simulink model "sim_2018"  (R2018a)
settings: Solver=ode4  StartTime=0.0  StopTime=31*60  FixedStep=0.001  RelTol=1e-3
model workspace: external: MAT-File E:\college\Sinior 2\2022\AutoPilot\task8\prameters.mat (data not in the file)
values from neighbouring files (symbols this model uses):
  g = aircraft_data(52)    [TF.m]    (also in param_code.m)
  IC = s0    [TF.m]    (also in param_code.m)
  Ixx = aircraft_data(53)    [TF.m]    (also in param_code.m)
  Iyy = aircraft_data(54)    [TF.m]    (also in param_code.m)
  Izz = aircraft_data(55)    [TF.m]    (also in param_code.m)
  m = aircraft_data(51)    [TF.m]    (also in param_code.m)
  mg0 = m*g * [ sin(s0(8)) ; -cos(s0(8))*sin(s0(7)) ; -cos(s0(8))*cos(s0(7)) ]    [TF.m]    (also in param_code.m)
  s0 = aircraft_data(4:15)    [TF.m]    (also in param_code.m)
  sdot0 = zeros(12,1)    [param_code.m]
  servo = tf(10,[1 10])    [TF.m]    (also in param_code.m)
  stability_matrix = [XU 0 XW 0 0 0 0 0 0 XDE XDTH;     0 U_Yv 0 Yp 0 Yr 0 U_Yda U_Ydr 0 0;     ZU 0 ZW 0 ZQ 0 ZWD 0 0 ZDE ZDTH;     0 U_Lv 0 U_Lp 0 U_Lr 0 U_Lda U_Ldr 0 0;     MU 0 MW 0 MQ 0 MWD 0 0 MDE MDTH;     0 U_Nv 0 U_Np 0 U_Nr 0 U_Nda U_Ndr 0 0]    [param_code.m]
  TH0 = s0(8)    [TF.m]    (also in param_code.m)
  U0 = s0(1)    [TF.m]    (also in param_code.m)
  W0 = s0(3)    [TF.m]    (also in param_code.m)
  z0 = s0(12)    [TF.m]    (also in param_code.m)
undefined symbols (not defined in the file or in its folder): rotationVectorToMatrix, sigbuilder_block
libraries: cstblocks x5, simulink_extras x3, shared6dof x1, sharedtransform x1, dspsigops x1
settings Model: Creator=engmh  LastModifiedBy=engmh

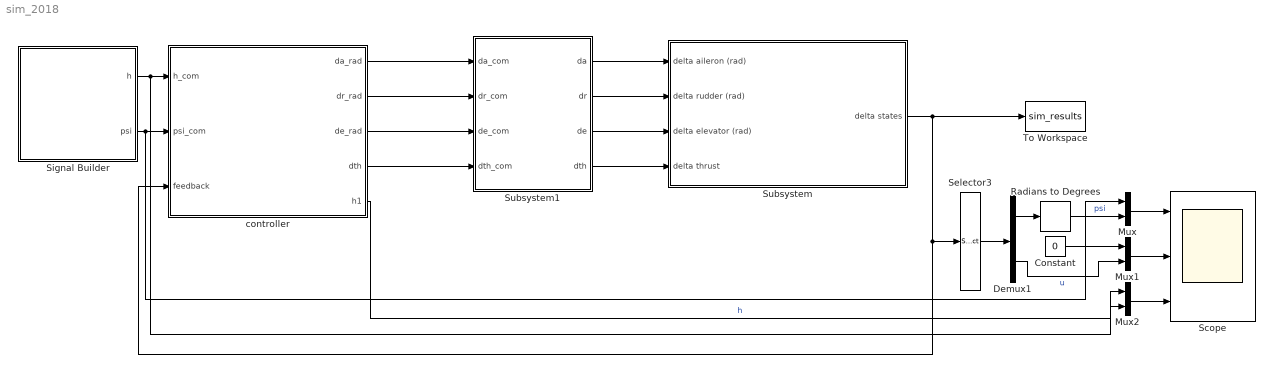
== system sim_2018 ==
  Constant : Constant  Value=0
  Demux1 : Demux  Outputs=2
  Mux : Mux  Inputs=2
  Mux1 : Mux  Inputs=2
  Mux2 : Mux  Inputs=2
  Radians to Degrees : simulink_extras/Transformations/Radians to Degrees
  Scope : Scope  NumInputPorts=3
  Selector3 : Selector  InputPortWidth=15  IndexOptions=Index vector (dialog)  Indices=[6 7 ]  OutputSizes=1
  Signal Builder : Subsystem  Tag=STV Subsys  LoadFcn=sigbuilder_block('load');  StartFcn=sigbuilder_block('start');  StopFcn=sigbuilder_block('stop');  ClipboardFcn=sigbuilder_block('clipboard');  mask(Sigbuilder block){tuvar=[0:10]}
      mask help: Simulink:masks:SigbuilderBlock_MD
      mask init:
      | if ~strcmp(get_param(bdroot(gcbh),'SimulationStatus'),'stopped') tuvar = sigbuilder_block('maskInit'); end
      settings: CopyFcn=sigbuilder_block('copy');  DeleteFcn=sigbuilder_block('delete');  ModelCloseFcn=sigbuilder_block('modelClose');  PreSaveFcn=sigbuilder_block('preSave');  PauseFcn=sigbuilder_block('pause');  ContinueFcn=sigbuilder_block('continue');  NameChangeFcn=sigbuilder_block('namechange');  OpenFcn=sigbuilder_block('open',[288.6 49.2 550.8 400.2 ]);  CloseFcn=sigbuilder_block('close');
      mask Display: plot(0, 0, 100, 100,[2, 2, 32, 32, 2], [68, 8, 8, 68, 68],[32, 2], [38, 38], [32, 19, 2],[53, 60, 44], [32, 17, 17, 2],[16, 16, 31, 31]);txt = getActiveGroup(gcbh);text(2, 100, txt,'verticalAlignment', 'top');
  Subsystem : Subsystem
  Subsystem1 : Subsystem
  To Workspace : ToWorkspace  VariableName=sim_results  SaveFormat=Timeseries  SampleTime=-1
  controller : Subsystem
  wires:
  Subsystem/1("delta states ") -> controller/3("feedback "), Selector3/1, To Workspace/1
  Subsystem1/1(da) -> Subsystem/1("delta aileron (rad) ")
  Subsystem1/2(dr) -> Subsystem/2(delta rudder (rad))
  Subsystem1/3(de) -> Subsystem/3(delta elevator (rad))
  Subsystem1/4(dth) -> Subsystem/4(delta thrust)
  Selector3/1 -> Demux1/1
  Demux1/1 -> Radians to Degrees/1
  Demux1/2 -> Mux1/2  "u"
  controller/1(da_rad) -> Subsystem1/1("da_com ")
  controller/2(dr_rad) -> Subsystem1/2(dr_com)
  controller/3(de_rad) -> Subsystem1/3(de_com)
  controller/4(dth) -> Subsystem1/4("dth_com ")
  controller/5("h1 ") -> Mux2/2  "h"
  Radians to Degrees/1 -> Mux/2  "psi"
  Signal Builder/2(psi) -> Mux/1, controller/2(psi_com)
  Signal Builder/1(h) -> Mux2/1, controller/1(h_com)
  Mux/1 -> Scope/1
  Mux1/1 -> Scope/2
  Mux2/1 -> Scope/3
  Constant/1 -> Mux1/1

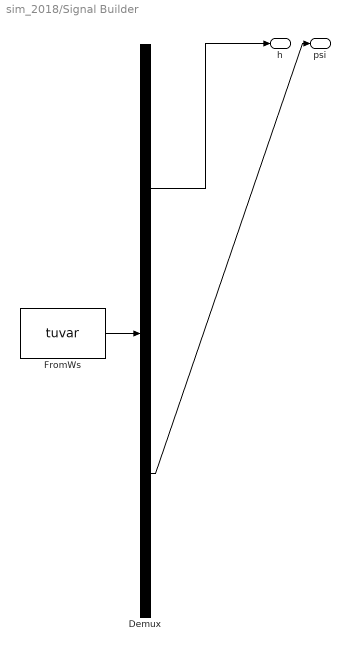
== system sim_2018/Signal Builder ==
  Demux : Demux  Tag=STV Demux  Outputs=2
  FromWs : FromWorkspace  Tag=STV FromWs  VariableName=tuvar  SampleTime=0
      SigBuilderData=|
      | common.afterFinalStr = 'Extrapolate'
      | common.sampleTime = 0
      | dataSet.timeRange = [0 1860]
      | dataSet.name = 'Group 1'
      | sbobj.Groups.Name = 'Group 1'
      | sbobj.Groups.Signals(1).Name = 'h'
      | sbobj.Groups.Signals(1).XData = [0 600 1080 1080 1200 1800 1860]
      | sbobj.Groups.Signals(1).YData = [0 10000 10000 10100 10100 0 0]
      | sbobj.Groups.Signals(2).Name = 'psi'
      | sbobj.Groups.Signals(2).XData = [0 720 720 1080 1080 1860]
      | sbobj.Groups.Signals(2).YData = [0 0 360 360 390 390]
      | sbobj.Groups.TimeRange = [0 1860]
  h : Outport  Tag=STV Outport
  psi : Outport  Tag=STV Outport  Port=2
  wires:
  Demux/1 -> h/1
  FromWs/1 -> Demux/1
  Demux/2 -> psi/1

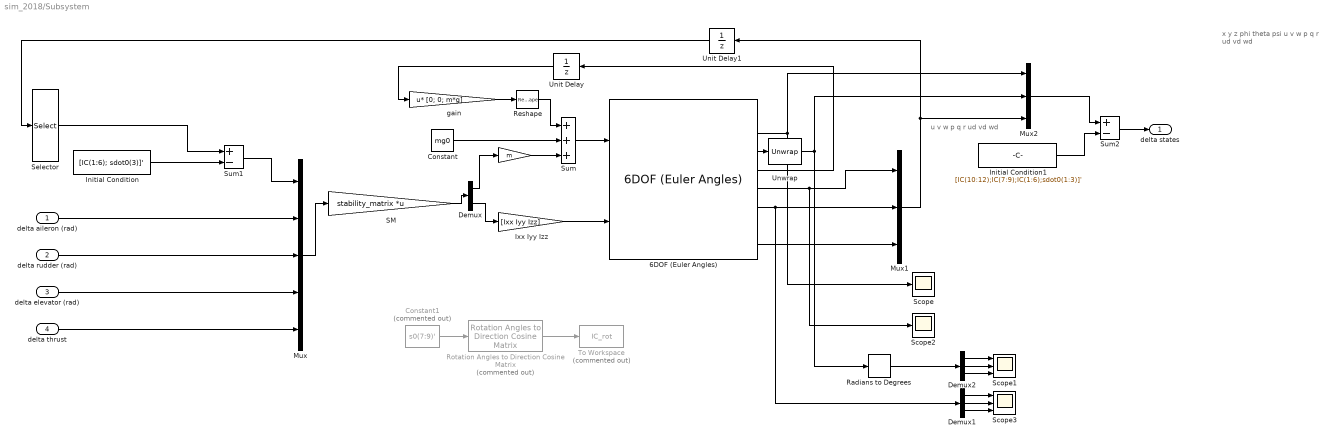
== system sim_2018/Subsystem ==
  note: u
      | v
      | w
      |
      | p
      | q
      | r
      |
      | ud
      | vd
      | wd
  note: x
      | y
      | z
      |
      | phi
      | theta
      | psi
      |
      | u
      | v
      | w
      |
      | p
      | q
      | r
      |
      | ud
      | vd
      | wd
  "delta aileron (rad) " : Inport
  delta rudder (rad) : Inport  Port=2
  delta elevator (rad) : Inport  Port=3
  delta thrust : Inport  Port=4
  " " : Gain  Gain=m
  6DOF (Euler Angles) : shared6dof/6DOF (Euler Angles)  units=English (Velocity in ft/s)  mtype=Fixed  rep=Euler Angles  xme_0=IC(10:12)'  Vm_0=IC(1:3)'  eul_0=IC(7:9)'  pm_0=IC(4:6)'  mass_0=m  mass_e=0.5  mass_f=2.0  inertia=I  inertia_e=eye(3)  inertia_f=2*eye(3)  k_quat=1.0  vre_flag=on  abi_flag=off  aMode=0
      settings: SourceProductBaseCode=AE,PW,DR,MT,UV,VE
  Constant : Constant  Value=mg0
  Constant1 : Constant  Commented=on  Value=s0(7:9)'
  Demux : Demux  Outputs=2
  Demux1 : Demux  Outputs=3
  Demux2 : Demux  Outputs=3
  Initial Condition : Constant  Value=[IC(1:6); sdot0(3)]'
  Initial Condition1 : Constant  Value=[IC(10:12);IC(7:9);IC(1:6);sdot0(1:3)]'
  Ixx Iyy Izz : Gain  Gain=[Ixx Iyy Izz]
  Mux : Mux  Inputs=5
  Mux1 : Mux  Inputs=3
  Mux2 : Mux  Inputs=3
  Radians to Degrees : simulink_extras/Transformations/Radians to Degrees
  Reshape : Reshape  OutputDimensionality=Row vector (2-D)
  Rotation Angles to Direction Cosine Matrix : sharedtransform/Rotation Angles to Direction Cosine Matrix  Commented=on  rotationOrder=ZYX  aMode=aMode
      settings: SourceProductBaseCode=AE,PW,DR,MT,UV,VE
  SM : Gain  Gain=stability_matrix  Multiplication=Matrix(K*u) (u vector)
  Scope : Scope
  Scope1 : Scope  NumInputPorts=3
  Scope2 : Scope
  Scope3 : Scope  NumInputPorts=3
  Selector : Selector  InputPortWidth=9  IndexOptions=Index vector (dialog)  Indices=[1:6 9]  OutputSizes=1
  Sum : Sum  Inputs=+++
  Sum1 : Sum  Inputs=+-
  Sum2 : Sum  Inputs=+-
  To Workspace : ToWorkspace  Commented=on  VariableName=IC_rot  SaveFormat=Timeseries  SampleTime=-1
  Unit Delay : UnitDelay  InitialCondition=rotationVectorToMatrix(IC(7:9))  SampleTime=-1
  Unit Delay1 : UnitDelay  InitialCondition=[IC(1:3); IC(4:6); sdot0(1:3)]'  SampleTime=-1
  Unwrap : dspsigops/Unwrap  tol=pi  running=off
  "gain " : Gain  Gain=[0; 0; m*g]  Multiplication=Matrix(u*K)
  "delta states " : Outport
  wires:
  Demux1/3 -> Scope3/3
  "delta aileron (rad) "/1 -> Mux/2
  " "/1 -> Sum/3
  Demux1/2 -> Scope3/2
  delta rudder (rad)/1 -> Mux/3
  Demux/2 -> Ixx Iyy Izz/1
  6DOF (Euler Angles)/5 -> Mux1/1, Scope2/1
  6DOF (Euler Angles)/2 -> Mux2/1, Scope/1
  Mux/1 -> SM/1
  Demux/1 -> " "/1
  Unwrap/1 -> Mux2/2, Radians to Degrees/1
  Ixx Iyy Izz/1 -> 6DOF (Euler Angles)/2
  Constant/1 -> Sum/2
  SM/1 -> Demux/1
  delta elevator (rad)/1 -> Mux/4
  Initial Condition/1 -> Sum1/2
  6DOF (Euler Angles)/4 -> Unit Delay/1
  Sum1/1 -> Mux/1
  Selector/1 -> Sum1/1
  6DOF (Euler Angles)/6 -> Demux1/1, Mux1/2
  "gain "/1 -> Reshape/1
  Sum/1 -> 6DOF (Euler Angles)/1
  Rotation Angles to Direction Cosine Matrix/1 -> To Workspace/1
  Constant1/1 -> Rotation Angles to Direction Cosine Matrix/1
  Demux1/1 -> Scope3/1
  Mux1/1 -> Mux2/3, Unit Delay1/1
  Reshape/1 -> Sum/1
  Unit Delay1/1 -> Selector/1
  Unit Delay/1 -> "gain "/1
  Demux2/1 -> Scope1/1
  Demux2/3 -> Scope1/3
  Demux2/2 -> Scope1/2
  delta thrust/1 -> Mux/5
  6DOF (Euler Angles)/8 -> Mux1/3
  Initial Condition1/1 -> Sum2/2
  Mux2/1 -> Sum2/1
  Sum2/1 -> "delta states "/1
  6DOF (Euler Angles)/3 -> Unwrap/1
  Radians to Degrees/1 -> Demux2/1

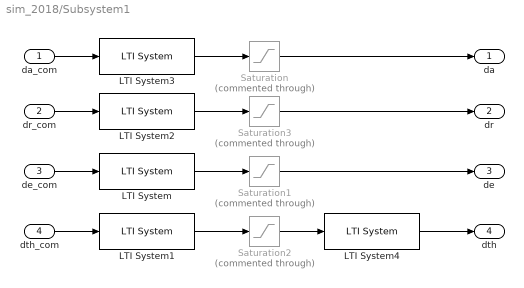
== system sim_2018/Subsystem1 ==
  "da_com " : Inport
  dr_com : Inport  Port=2
  de_com : Inport  Port=3
  "dth_com " : Inport  Port=4
  LTI System : cstblocks/LTI System  sys=-servo  IC=[]
  LTI System1 : cstblocks/LTI System  sys=servo  IC=[]
  LTI System2 : cstblocks/LTI System  sys=servo  IC=[]
  LTI System3 : cstblocks/LTI System  sys=servo  IC=[]
  LTI System4 : cstblocks/LTI System  sys=engine_timelag  IC=[]
  Saturation{,1..3} (4 alike) : Saturate  Commented=through
  da : Outport
  dr : Outport  Port=2
  de : Outport  Port=3
  dth : Outport  Port=4
  wires:
  "dth_com "/1 -> LTI System1/1
  Saturation2/1 -> LTI System4/1
  LTI System2/1 -> Saturation3/1
  LTI System3/1 -> Saturation/1
  de_com/1 -> LTI System/1
  LTI System1/1 -> Saturation2/1
  Saturation1/1 -> de/1
  LTI System/1 -> Saturation1/1
  dr_com/1 -> LTI System2/1
  Saturation/1 -> da/1
  "da_com "/1 -> LTI System3/1
  LTI System4/1 -> dth/1
  Saturation3/1 -> dr/1

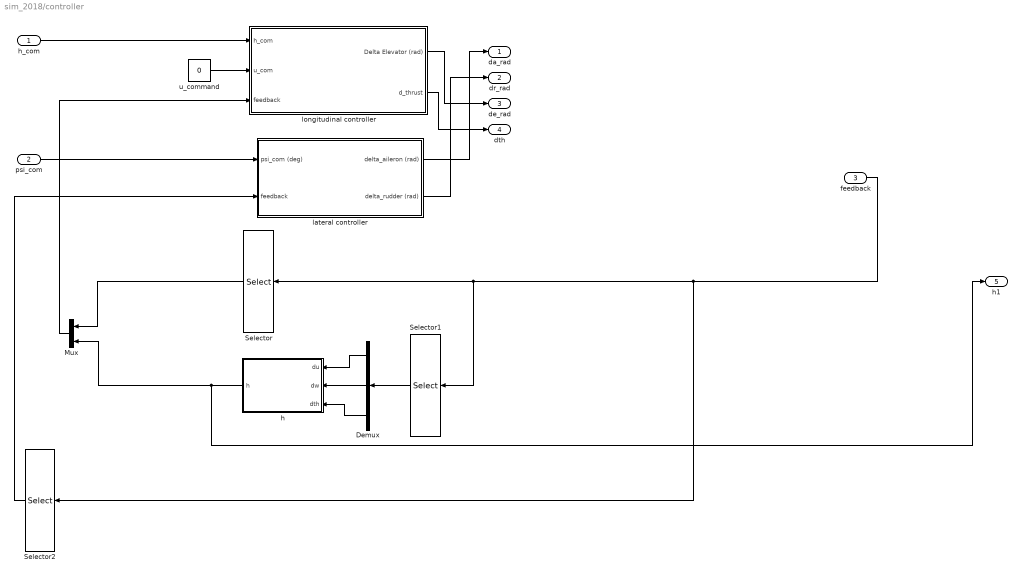
== system sim_2018/controller ==
  h_com : Inport
  psi_com : Inport  Port=2
  "feedback " : Inport  Port=3
  Demux : Demux  Outputs=3
  Mux : Mux  Inputs=2
  Selector : Selector  InputPortWidth=15  IndexOptions=Index vector (dialog)  Indices=[11 5 7]  OutputSizes=1
  Selector1 : Selector  InputPortWidth=15  IndexOptions=Index vector (dialog)  Indices=[7 9 5]  OutputSizes=1
  Selector2 : Selector  InputPortWidth=15  IndexOptions=Index vector (dialog)  Indices=[4 6 12]  OutputSizes=1
  h : Subsystem
  lateral controller : Subsystem
  longitudinal controller : Subsystem
  u_command : Constant  Value=0
  da_rad : Outport
  dr_rad : Outport  Port=2
  de_rad : Outport  Port=3
  dth : Outport  Port=4
  "h1 " : Outport  Port=5
  wires:
  h/1("h ") -> "h1 "/1, Mux/2
  Demux/1 -> h/1(du)
  "feedback "/1 -> Selector1/1, Selector/1, Selector2/1
  Demux/3 -> h/3(dth)
  Demux/2 -> h/2(dw)
  Selector/1 -> Mux/1
  Mux/1 -> longitudinal controller/3("feedback ")
  Selector1/1 -> Demux/1
  h_com/1 -> longitudinal controller/1(h_com)
  longitudinal controller/1(Delta Elevator (rad)) -> de_rad/1
  lateral controller/2(delta_rudder (rad)) -> dr_rad/1
  u_command/1 -> longitudinal controller/2(u_com)
  Selector2/1 -> lateral controller/2(feedback)
  psi_com/1 -> lateral controller/1(psi_com (deg))
  longitudinal controller/2(d_thrust) -> dth/1
  lateral controller/1(delta_aileron (rad)) -> da_rad/1

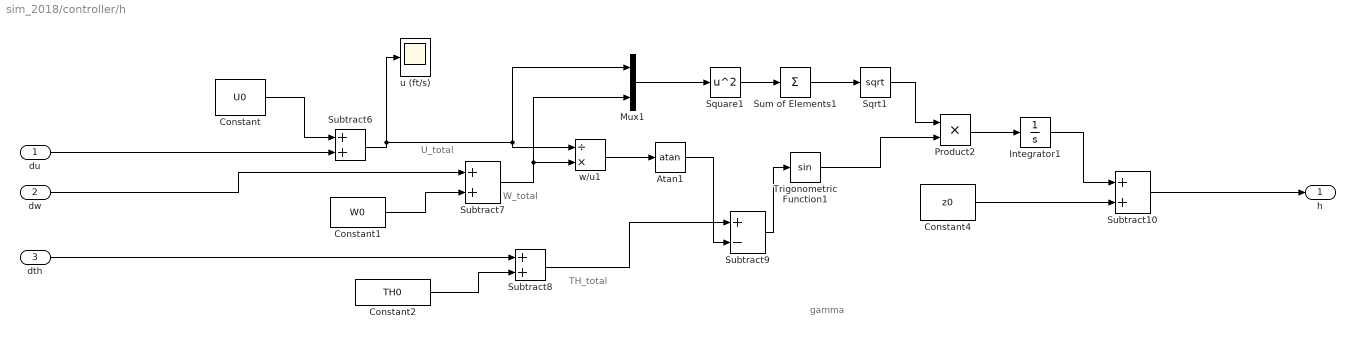
== system sim_2018/controller/h ==
  note: U_total
  note: W_total
  note: TH_total
  note: gamma
  du : Inport
  dw : Inport  Port=2
  dth : Inport  Port=3
  Atan1 : Trigonometry  Operator=atan
  Constant : Constant  Value=U0
  Constant1 : Constant  Value=W0
  Constant2 : Constant  Value=TH0  VectorParams1D=off
  Constant4 : Constant  Value=z0
  Integrator1 : Integrator
  Mux1 : Mux  Inputs=2
  Product2 : Product
  Sqrt1 : Sqrt  SaturateOnIntegerOverflow=on
  Square1 : Math  Operator=square  SaturateOnIntegerOverflow=on
  Subtract{6..8,10} (4 alike) : Sum
  Subtract9 : Sum  Inputs=+-
  Sum of Elements1 : Sum  Inputs=+
  Trigonometric Function1 : Trigonometry
  u (ft/s) : Scope
  w/u1 : Product  Inputs=/*
  "h " : Outport
  wires:
  Constant4/1 -> Subtract10/2
  w/u1/1 -> Atan1/1
  Subtract7/1 -> w/u1/2, Mux1/2
  Constant1/1 -> Subtract7/2
  Square1/1 -> Sum of Elements1/1
  Subtract8/1 -> Subtract9/1
  Constant/1 -> Subtract6/1
  Subtract9/1 -> Trigonometric Function1/1
  Sum of Elements1/1 -> Sqrt1/1
  Trigonometric Function1/1 -> Product2/2
  Constant2/1 -> Subtract8/2
  du/1 -> Subtract6/2
  dth/1 -> Subtract8/1
  Sqrt1/1 -> Product2/1
  dw/1 -> Subtract7/1
  Subtract6/1 -> u (ft/s)/1, w/u1/1, Mux1/1
  Integrator1/1 -> Subtract10/1
  Mux1/1 -> Square1/1
  Product2/1 -> Integrator1/1
  Atan1/1 -> Subtract9/2
  Subtract10/1 -> "h "/1

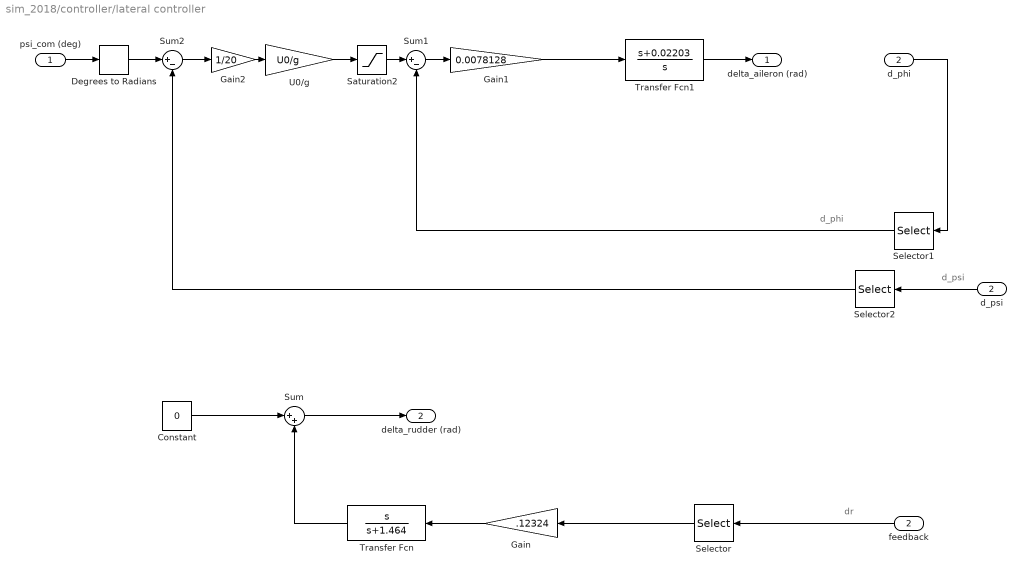
== system sim_2018/controller/lateral controller ==
  note: dr
  note: d_psi
  note: d_phi
  psi_com (deg) : Inport
  feedback : Inport  Port=2
  Constant : Constant  Value=0
  Degrees to Radians : simulink_extras/Transformations/Degrees to Radians
  Gain : Gain  Gain=.12324
  Gain1 : Gain  Gain=0.0078128
  Gain2 : Gain  Gain=1/20
  Saturation2 : Saturate  UpperLimit=30*pi/180  LowerLimit=-30*pi/180
  Selector : Selector  InputPortWidth=3  IndexOptions=Index vector (dialog)  Indices=[3]  OutputSizes=1
  Selector1 : Selector  InputPortWidth=3  IndexOptions=Index vector (dialog)  Indices=[1]  OutputSizes=1
  Selector2 : Selector  InputPortWidth=3  IndexOptions=Index vector (dialog)  Indices=[2]  OutputSizes=1
  Sum : Sum  Inputs=|++
  Sum1 : Sum  Inputs=|+-
  Sum2 : Sum  Inputs=|+-
  Transfer Fcn : TransferFcn  Numerator=[1 0]  Denominator=[1 1.464]
  Transfer Fcn1 : TransferFcn  Numerator=[1 0.02203]  Denominator=[1 0]
  U0/g : Gain  Gain=U0/g
  d_phi : InportShadow  Port=2
  d_psi : InportShadow  Port=2
  delta_aileron (rad) : Outport  VectorParamsAs1DForOutWhenUnconnected=on
  delta_rudder (rad) : Outport  Port=2  VectorParamsAs1DForOutWhenUnconnected=on
  wires:
  Degrees to Radians/1 -> Sum2/1
  Selector/1 -> Gain/1
  psi_com (deg)/1 -> Degrees to Radians/1
  Gain/1 -> Transfer Fcn/1
  Transfer Fcn1/1 -> delta_aileron (rad)/1
  Selector1/1 -> Sum1/2
  Sum/1 -> delta_rudder (rad)/1
  U0/g/1 -> Saturation2/1
  Sum2/1 -> Gain2/1
  Sum1/1 -> Gain1/1
  Transfer Fcn/1 -> Sum/2
  Gain2/1 -> U0/g/1
  feedback/1 -> Selector/1
  Gain1/1 -> Transfer Fcn1/1
  Selector2/1 -> Sum2/2
  Saturation2/1 -> Sum1/1
  d_phi/1 -> Selector1/1
  Constant/1 -> Sum/1
  d_psi/1 -> Selector2/1

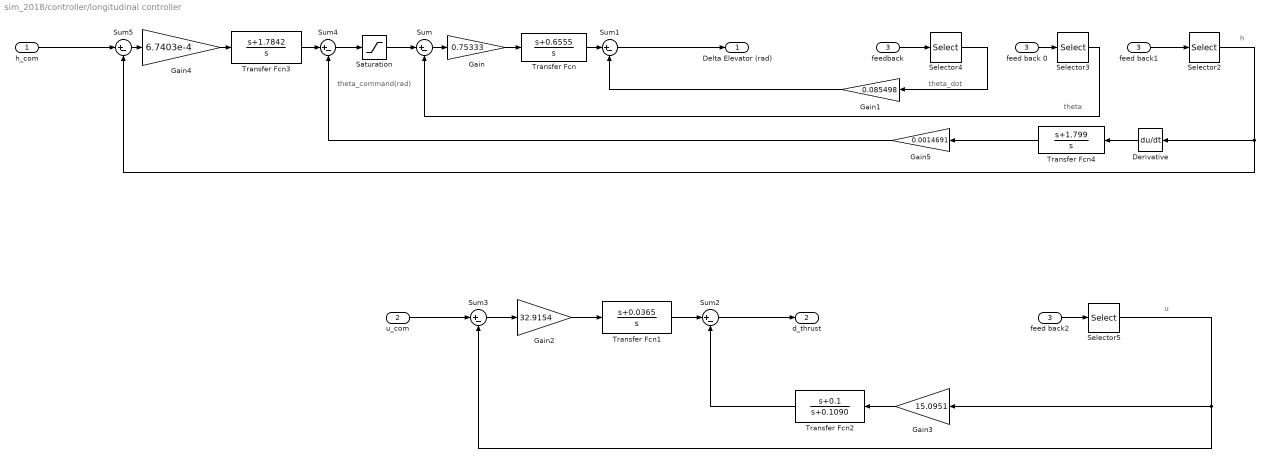
== system sim_2018/controller/longitudinal controller ==
  note: u
  note: theta
  note: theta_command(rad)
  note: theta_dot
  note: h
  h_com : Inport
  u_com : Inport  Port=2
  "feedback " : Inport  Port=3
  Derivative : Derivative
  Gain : Gain  Gain=0.75333
  Gain1 : Gain  Gain=0.085498
  Gain2 : Gain  Gain=32.9154
  Gain3 : Gain  Gain=15.0951
  Gain4 : Gain  Gain=6.7403e-4
  Gain5 : Gain  Gain=0.0014691
  Saturation : Saturate  LowerLimit=-.5
  Selector2 : Selector  InputPortWidth=4  IndexOptions=Index vector (dialog)  Indices=[4]  OutputSizes=1
  Selector3 : Selector  InputPortWidth=4  IndexOptions=Index vector (dialog)  Indices=[2]  OutputSizes=1
  Selector4 : Selector  InputPortWidth=4  IndexOptions=Index vector (dialog)  Indices=[1]  OutputSizes=1
  Selector5 : Selector  InputPortWidth=4  IndexOptions=Index vector (dialog)  Indices=[3]  OutputSizes=1
  Sum{,1..5} (6 alike) : Sum  Inputs=|+-
  Transfer Fcn : TransferFcn  Numerator=[1 +0.6555]  Denominator=[1 0]
  Transfer Fcn1 : TransferFcn  Numerator=[1 0.0365]  Denominator=[1 0]
  Transfer Fcn2 : TransferFcn  Numerator=[1 0.1]  Denominator=[1 0.1090]
  Transfer Fcn3 : TransferFcn  Numerator=[1 1.7842]  Denominator=[1 0]
  Transfer Fcn4 : TransferFcn  Numerator=[1 +1.799]  Denominator=[1 0]
  "feed back 0 " : InportShadow  Port=3
  feed back1 : InportShadow  Port=3
  feed back2 : InportShadow  Port=3
  Delta Elevator (rad) : Outport  VectorParamsAs1DForOutWhenUnconnected=on
  d_thrust : Outport  Port=2  VectorParamsAs1DForOutWhenUnconnected=on
  wires:
  Gain2/1 -> Transfer Fcn1/1
  Selector4/1 -> Gain1/1
  Gain/1 -> Transfer Fcn/1
  "feed back 0 "/1 -> Selector3/1
  Sum5/1 -> Gain4/1
  Selector2/1 -> Derivative/1, Sum5/2
  Sum/1 -> Gain/1
  Transfer Fcn/1 -> Sum1/1
  Sum4/1 -> Saturation/1
  Selector5/1 -> Gain3/1, Sum3/2
  Derivative/1 -> Transfer Fcn4/1
  Selector3/1 -> Sum/2
  feed back1/1 -> Selector2/1
  Transfer Fcn2/1 -> Sum2/2
  Transfer Fcn1/1 -> Sum2/1
  Transfer Fcn3/1 -> Sum4/1
  Saturation/1 -> Sum/1
  Gain3/1 -> Transfer Fcn2/1
  Sum1/1 -> Delta Elevator (rad)/1
  Gain5/1 -> Sum4/2
  u_com/1 -> Sum3/1
  h_com/1 -> Sum5/1
  Gain1/1 -> Sum1/2
  Sum3/1 -> Gain2/1
  Transfer Fcn4/1 -> Gain5/1
  Gain4/1 -> Transfer Fcn3/1
  feed back2/1 -> Selector5/1
  "feedback "/1 -> Selector4/1
  Sum2/1 -> d_thrust/1
